simulink model "StateObserver_4"  (Simulink 8.3)
settings: configuration reference "mpc555rt_ref_debug_config" (kept outside this file)
values from neighbouring files (symbols this model uses):
  dt = 0.0192307692308    [newvars_4_25.mat]
  g = 32.174    [newvars_4_25.mat]
  HD0noaa = 48.3774    [newvars_4_25.mat]
  HE0noaa = 0.8962    [newvars_4_25.mat]
  HN0noaa = 20.6483    [newvars_4_25.mat]
  P0_est_sta = [100 0 0 0 0 0 0 0 0 0 0 0 ... (225 elements, 15x15)]    [newvars_4_25.mat]
  Q_obs_sta = [0.001 0 0 0 0 0 0 0 0 0 0 0 ... (225 elements, 15x15)]    [newvars_4_25.mat]
  R_obs_sta = [1 0 0 0 0 0 0 0 0 0 0.01 0 ... (81 elements, 9x9)]    [newvars_4_25.mat]
  saturation_max_sta = [1 0.261799387799 0.349065850399 0.174532925199 200 1.57079632679 1.57079632679 3.14159265359 3.14159265359 inf 15.7079632679 15.7079632679 ... (15 elements, 1x15)]    [newvars_4_25.mat]
  saturation_min_sta = [0.15 -0.261799387799 -0.349065850399 -0.174532925199 2.22044604925e-15 -1.57079632679 -1.57079632679 -3.14159265359 -3.14159265359 -inf -15.7079632679 -15.7079632679 ... (15 elements, 1x15)]    [newvars_4_25.mat]
  x0_est_sta = [0.55 0.0200712863979 0 0 45.808269954 -0.00604049793249 0 0 -0.00232644648767 0 0 -6.36434657562e-08 ... (15 elements, 15x1)]    [newvars_4_25.mat]
settings Model: Creator=Rick Riley  LastModifiedBy=gonzalo
settings ConfigSet: SourceName=mpc555rt_ref_debug_config  SourceLocation=Base Workspace

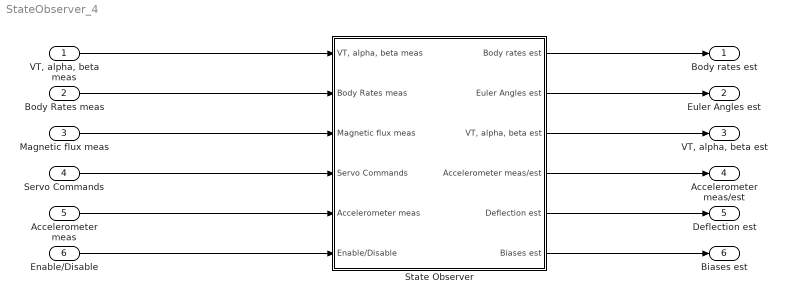
== system StateObserver_4 ==
  "VT, alpha, beta meas" : Inport  OutDataTypeStr=Bus: VT_A_B_bus  SampleTime=dt  BusOutputAsStruct=on
  Body Rates meas : Inport  Port=2  OutDataTypeStr=Bus: INS_rates_bus  SampleTime=dt
  Magnetic flux meas : Inport  Port=3  OutDataTypeStr=Bus: MagnetometerFlux
  Servo Commands : Inport  Port=4  OutDataTypeStr=Bus: Control_cmd_bus
  Accelerometer meas : Inport  Port=5  OutDataTypeStr=Bus: Accelerometer
  Enable/Disable : Inport  Port=6  OutDataTypeStr=boolean  SampleTime=dt
  State Observer : Subsystem
  Body rates est : Outport  OutDataTypeStr=Bus: INS_rates_bus  BusOutputAsStruct=on
  Euler Angles est : Outport  Port=2  OutDataTypeStr=Bus: INS_angles_bus  BusOutputAsStruct=on
  "VT, alpha, beta est" : Outport  Port=3  OutDataTypeStr=Bus: VT_A_B_bus  BusOutputAsStruct=on
  Accelerometer meas/est : Outport  Port=4  OutDataTypeStr=Bus: Accelerometer  BusOutputAsStruct=on
  Deflection est : Outport  Port=5  OutDataTypeStr=Bus: ControlSurfaceDeflections  BusOutputAsStruct=on
  Biases est : Outport  Port=6  BusOutputAsStruct=on
  wires:
  "VT, alpha, beta meas"/1 -> State Observer/1("VT, alpha, beta meas")
  Body Rates meas/1 -> State Observer/2(Body Rates meas)
  State Observer/3("VT, alpha, beta est") -> "VT, alpha, beta est"/1
  State Observer/1(Body rates est) -> Body rates est/1
  State Observer/2(Euler Angles est) -> Euler Angles est/1
  State Observer/4(Accelerometer meas/est) -> Accelerometer meas/est/1
  Enable/Disable/1 -> State Observer/6(Enable/Disable)
  State Observer/5(Deflection est) -> Deflection est/1
  State Observer/6(Biases est) -> Biases est/1
  Magnetic flux meas/1 -> State Observer/3(Magnetic flux meas)
  Servo Commands/1 -> State Observer/4(Servo Commands)
  Accelerometer meas/1 -> State Observer/5(Accelerometer meas)

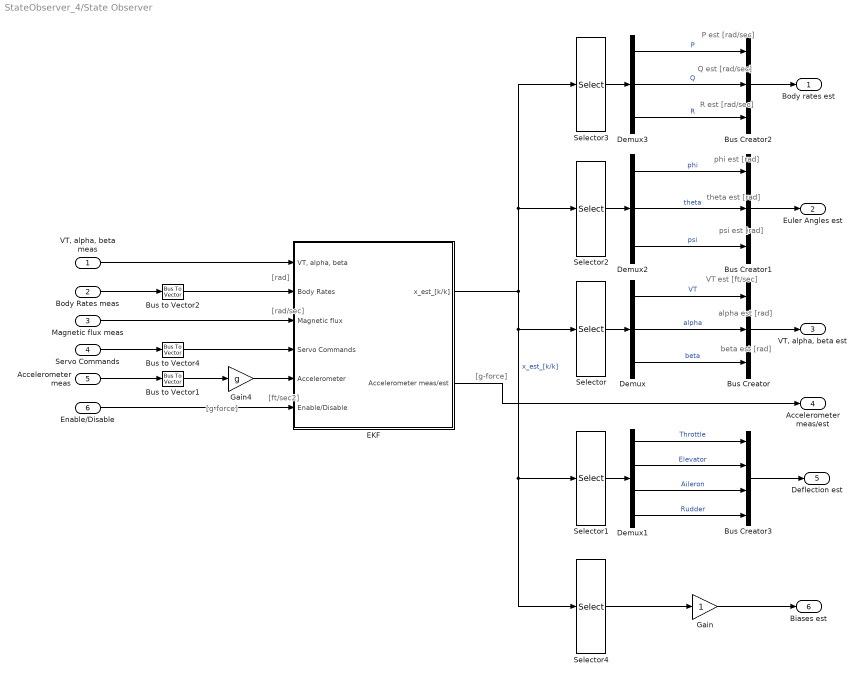
== system StateObserver_4/State Observer ==
  note: alpha est [rad]
  note: beta est [rad]
  note: VT est [ft/sec]
  note: Q est [rad/sec]
  note: R est [rad/sec]
  note: P est [rad/sec]
  note: phi est [rad]
  note: theta est [rad]
  note: [ft/sec2]
  note: [g-force]
  note: [rad/sec]
  note: [rad]
  note: psi est [rad]
  note: [g-force]
  "VT, alpha, beta meas" : Inport
  Body Rates meas : Inport  Port=2  OutDataTypeStr=Bus: INS_rates_bus  SampleTime=dt
  Magnetic flux meas : Inport  Port=3  OutDataTypeStr=Bus: MagnetometerFlux
  Servo Commands : Inport  Port=4  OutDataTypeStr=Bus: Control_cmd_bus  BusOutputAsStruct=on
  Accelerometer meas : Inport  Port=5  OutDataTypeStr=Bus: Accelerometer
  Enable/Disable : Inport  Port=6  OutDataTypeStr=boolean  SampleTime=dt
  Bus Creator : BusCreator  Inputs=3  OutDataTypeStr=Bus: VT_A_B_bus  NonVirtualBus=on
  Bus Creator1 : BusCreator  Inputs=3  OutDataTypeStr=Bus: INS_angles_bus  NonVirtualBus=on
  Bus Creator2 : BusCreator  Inputs=3  OutDataTypeStr=Bus: INS_rates_bus  NonVirtualBus=on
  Bus Creator3 : BusCreator  OutDataTypeStr=Bus: ControlSurfaceDeflections  NonVirtualBus=on
  Bus to Vector1 : BusToVector
  Bus to Vector2 : BusToVector
  Bus to Vector4 : BusToVector
  Demux : Demux  Outputs=3
  Demux1 : Demux
  Demux2 : Demux  Outputs=3
  Demux3 : Demux  Outputs=3
  EKF : Subsystem
  Gain : Gain
  Gain4 : Gain  Gain=g
  Selector : Selector  InputPortWidth=15  Indices=[5 6 7]
  Selector1 : Selector  InputPortWidth=15  Indices=[1 2 3 4]
  Selector2 : Selector  InputPortWidth=15  Indices=[8 9 10]
  Selector3 : Selector  InputPortWidth=15  Indices=[11 12 13]
  Selector4 : Selector  InputPortWidth=15  Indices=[14 15]
  Body rates est : Outport  OutDataTypeStr=Bus: INS_rates_bus
  Euler Angles est : Outport  Port=2  OutDataTypeStr=Bus: INS_angles_bus  BusOutputAsStruct=on
  "VT, alpha, beta est" : Outport  Port=3  OutDataTypeStr=Bus: VT_A_B_bus
  Accelerometer meas/est : Outport  Port=4  OutDataTypeStr=Bus: Accelerometer  BusOutputAsStruct=on
  Deflection est : Outport  Port=5  OutDataTypeStr=Bus: ControlSurfaceDeflections  BusOutputAsStruct=on
  Biases est : Outport  Port=6  BusOutputAsStruct=on
  wires:
  Bus Creator/1 -> "VT, alpha, beta est"/1
  Demux/1 -> Bus Creator/1  "VT"
  Demux/2 -> Bus Creator/2  "alpha"
  Demux/3 -> Bus Creator/3  "beta"
  Selector/1 -> Demux/1
  Selector2/1 -> Demux2/1
  Demux2/1 -> Bus Creator1/1  "phi"
  Demux2/2 -> Bus Creator1/2  "theta"
  Bus Creator1/1 -> Euler Angles est/1
  Bus Creator2/1 -> Body rates est/1
  Demux3/1 -> Bus Creator2/1  "P"
  Demux3/2 -> Bus Creator2/2  "Q"
  Demux3/3 -> Bus Creator2/3  "R"
  Selector3/1 -> Demux3/1
  Bus to Vector1/1 -> Gain4/1
  Accelerometer meas/1 -> Bus to Vector1/1
  Body Rates meas/1 -> Bus to Vector2/1
  Bus to Vector2/1 -> EKF/2(Body Rates)
  Gain4/1 -> EKF/5(Accelerometer)
  "VT, alpha, beta meas"/1 -> EKF/1("VT, alpha, beta")
  Servo Commands/1 -> Bus to Vector4/1
  Demux2/3 -> Bus Creator1/3  "psi"
  EKF/2(Accelerometer meas/est) -> Accelerometer meas/est/1
  Enable/Disable/1 -> EKF/6(Enable/Disable)
  Selector1/1 -> Demux1/1
  Demux1/4 -> Bus Creator3/4  "Rudder"
  Demux1/2 -> Bus Creator3/2  "Elevator"
  Demux1/3 -> Bus Creator3/3  "Aileron"
  Demux1/1 -> Bus Creator3/1  "Throttle"
  Bus Creator3/1 -> Deflection est/1
  EKF/1(x_est_[k/k]) -> Selector3/1, Selector2/1, Selector/1, Selector1/1, Selector4/1  "x_est_[k/k]"
  Selector4/1 -> Gain/1
  Gain/1 -> Biases est/1
  Magnetic flux meas/1 -> EKF/3(Magnetic flux)
  Bus to Vector4/1 -> EKF/4(Servo Commands)

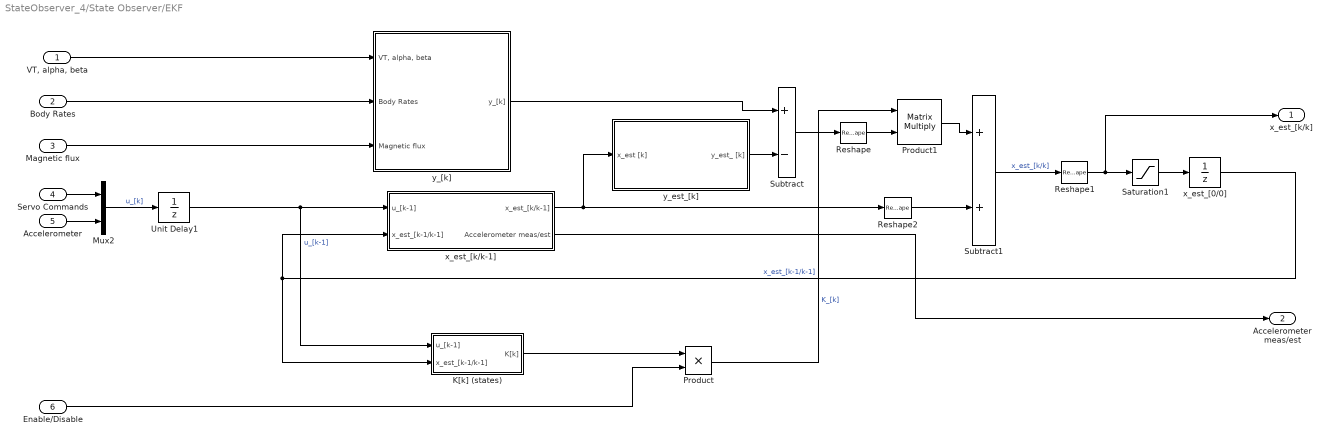
== system StateObserver_4/State Observer/EKF ==
  "VT, alpha, beta" : Inport  OutDataTypeStr=Bus: VT_A_B_bus
  Body Rates : Inport  Port=2  SampleTime=dt
  Magnetic flux : Inport  Port=3  OutDataTypeStr=Bus: MagnetometerFlux
  Servo Commands : Inport  Port=4
  Accelerometer : Inport  Port=5
  Enable/Disable : Inport  Port=6  OutDataTypeStr=boolean  SampleTime=dt
  K[k] (states) : Subsystem
  Mux2 : Mux  Inputs=2
  Product : Product  RndMeth=Zero
  Product1 : Product  Multiplication=Matrix(*)  RndMeth=Zero
  Reshape : Reshape  OutputDimensionality=Column vector (2-D)
  Reshape1 : Reshape
  Reshape2 : Reshape  OutputDimensionality=Column vector (2-D)
  Saturation1 : Saturate  UpperLimit=saturation_max_sta  LowerLimit=saturation_min_sta
  Subtract : Sum  Inputs=+-
  Subtract1 : Sum
  Unit Delay1 : UnitDelay  SampleTime=dt
  x_est_[0/0] : UnitDelay  InitialCondition=x0_est_sta  SampleTime=dt
  x_est_[k/k-1] : Subsystem
  y_[k] : Subsystem
  y_est_[k] : Subsystem
  x_est_[k/k] : Outport
  Accelerometer meas/est : Outport  Port=2  OutDataTypeStr=Bus: Accelerometer  BusOutputAsStruct=on
  wires:
  y_[k]/1(y_[k]) -> Subtract/1
  "VT, alpha, beta"/1 -> y_[k]/1("VT, alpha, beta")
  Subtract1/1 -> Reshape1/1  "x_est_[k/k]"
  x_est_[0/0]/1 -> K[k] (states)/2(x_est_[k-1/k-1]), x_est_[k/k-1]/2(x_est_[k-1/k-1])  "x_est_[k-1/k-1]"
  Unit Delay1/1 -> K[k] (states)/1(u_[k-1]), x_est_[k/k-1]/1(u_[k-1])  "u_[k-1]"
  Saturation1/1 -> x_est_[0/0]/1
  y_est_[k]/1(y_est_ [k]) -> Subtract/2
  Product/1 -> Product1/1  "K_[k]"
  Product1/1 -> Subtract1/1
  Mux2/1 -> Unit Delay1/1  "u_[k]"
  Accelerometer/1 -> Mux2/2
  Servo Commands/1 -> Mux2/1
  Body Rates/1 -> y_[k]/2(Body Rates)
  Subtract/1 -> Reshape/1
  x_est_[k/k-1]/1(x_est_[k/k-1]) -> Reshape2/1, y_est_[k]/1(x_est [k])
  x_est_[k/k-1]/2(Accelerometer meas/est) -> Accelerometer meas/est/1
  K[k] (states)/1(K[k]) -> Product/1
  Enable/Disable/1 -> Product/2
  Reshape/1 -> Product1/2
  Reshape1/1 -> Saturation1/1, x_est_[k/k]/1
  Reshape2/1 -> Subtract1/2
  Magnetic flux/1 -> y_[k]/3(Magnetic flux)

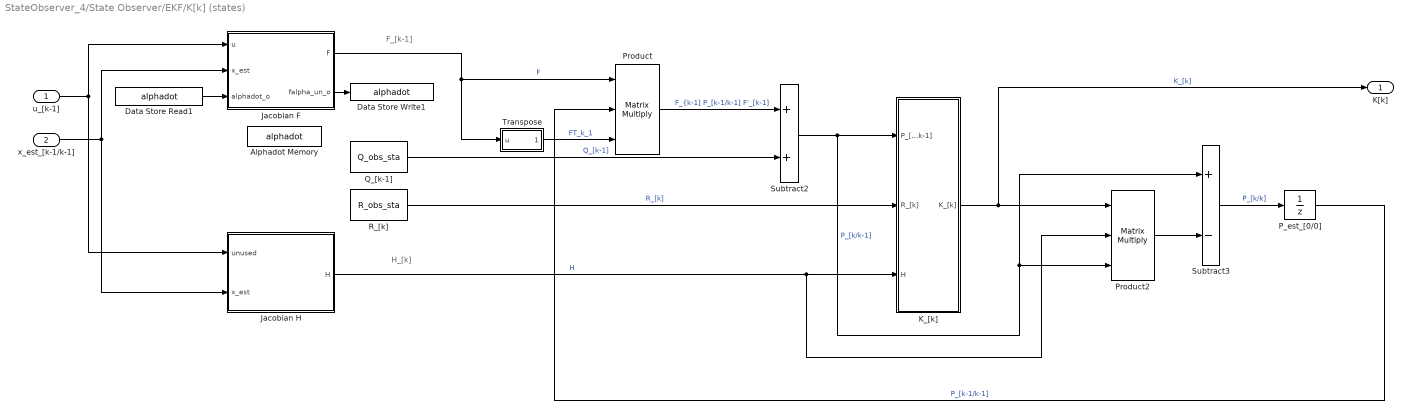
== system StateObserver_4/State Observer/EKF/K[k] (states) ==
  note: H_[k]
  note: F_[k-1]
  u_[k-1] : Inport
  x_est_[k-1/k-1] : Inport  Port=2
  Alphadot Memory : DataStoreMemory  DataStoreName=alphadot  ReadBeforeWriteMsg=warning  WriteAfterWriteMsg=warning  WriteAfterReadMsg=warning  OutDataTypeStr=double
  Data Store Read1 : DataStoreRead  DataStoreName=alphadot  SampleTime=dt
  Data Store Write1 : DataStoreWrite  DataStoreName=alphadot
  Jacobian F : MATLAB Function  TreatAsAtomicUnit=on
  Jacobian H : MATLAB Function  TreatAsAtomicUnit=on
  K_[k] : Subsystem
  P_est_[0/0] : UnitDelay  InitialCondition=P0_est_sta  SampleTime=dt
  Product : Product  Inputs=3  Multiplication=Matrix(*)  RndMeth=Zero
  Product2 : Product  Inputs=3  Multiplication=Matrix(*)  RndMeth=Zero
  Q_[k-1] : Constant  Value=Q_obs_sta
  R_[k] : Constant  Value=R_obs_sta
  Subtract2 : Sum
  Subtract3 : Sum  Inputs=+-
  Transpose : MATLAB Function  TreatAsAtomicUnit=on
  K[k] : Outport
  wires:
  K_[k]/1(K_[k]) -> K[k]/1, Product2/1  "K_[k]"
  x_est_[k-1/k-1]/1 -> Jacobian F/2(x_est), Jacobian H/2(x_est)
  u_[k-1]/1 -> Jacobian F/1(u), Jacobian H/1(unused)
  Jacobian F/1(F) -> Transpose/1(u), Product/1  "F"
  P_est_[0/0]/1 -> Product/2  "P_[k-1/k-1]"
  Subtract3/1 -> P_est_[0/0]/1  "P_[k/k]"
  Product2/1 -> Subtract3/2
  R_[k]/1 -> K_[k]/2(R_[k])  "R_[k]"
  Jacobian H/1(H) -> Product2/2, K_[k]/3(H)  "H"
  Subtract2/1 -> Product2/3, Subtract3/1, K_[k]/1(P_[k/k-1])  "P_[k/k-1]"
  Q_[k-1]/1 -> Subtract2/2  "Q_[k-1]"
  Product/1 -> Subtract2/1  "F_{k-1] P_[k-1/k-1] F'_[k-1]"
  Transpose/1(FT_k_1) -> Product/3  "FT_k_1"
  Data Store Read1/1 -> Jacobian F/3(alphadot_o)
  Jacobian F/2(falpha_un_o) -> Data Store Write1/1

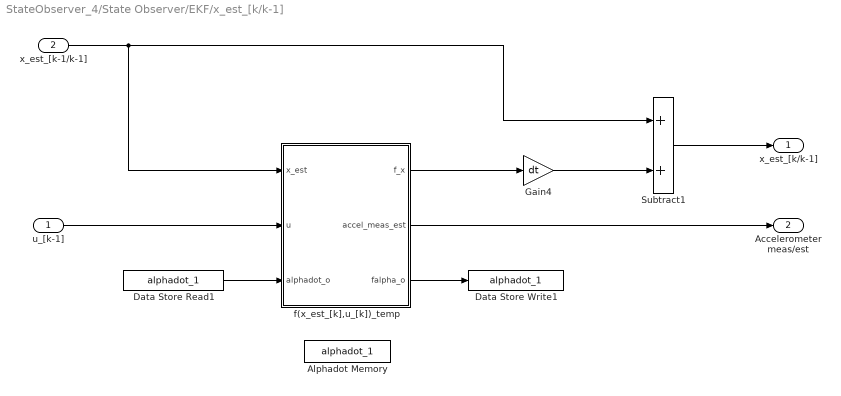
== system StateObserver_4/State Observer/EKF/x_est_[k/k-1] ==
  u_[k-1] : Inport
  x_est_[k-1/k-1] : Inport  Port=2
  Alphadot Memory : DataStoreMemory  DataStoreName=alphadot_1  ReadBeforeWriteMsg=warning  WriteAfterWriteMsg=warning  WriteAfterReadMsg=warning  OutDataTypeStr=double
  Data Store Read1 : DataStoreRead  DataStoreName=alphadot_1  SampleTime=dt
  Data Store Write1 : DataStoreWrite  DataStoreName=alphadot_1
  Gain4 : Gain  Gain=dt
  Subtract1 : Sum
  f(x_est_[k],u_[k])_temp : MATLAB Function  TreatAsAtomicUnit=on
  x_est_[k/k-1] : Outport
  Accelerometer meas/est : Outport  Port=2  OutDataTypeStr=Bus: Accelerometer  BusOutputAsStruct=on
  wires:
  Gain4/1 -> Subtract1/2
  x_est_[k-1/k-1]/1 -> Subtract1/1, f(x_est_[k],u_[k])_temp/1(x_est)
  u_[k-1]/1 -> f(x_est_[k],u_[k])_temp/2(u)
  Subtract1/1 -> x_est_[k/k-1]/1
  f(x_est_[k],u_[k])_temp/1(f_x) -> Gain4/1
  f(x_est_[k],u_[k])_temp/2(accel_meas_est) -> Accelerometer meas/est/1
  f(x_est_[k],u_[k])_temp/3(falpha_o) -> Data Store Write1/1
  Data Store Read1/1 -> f(x_est_[k],u_[k])_temp/3(alphadot_o)

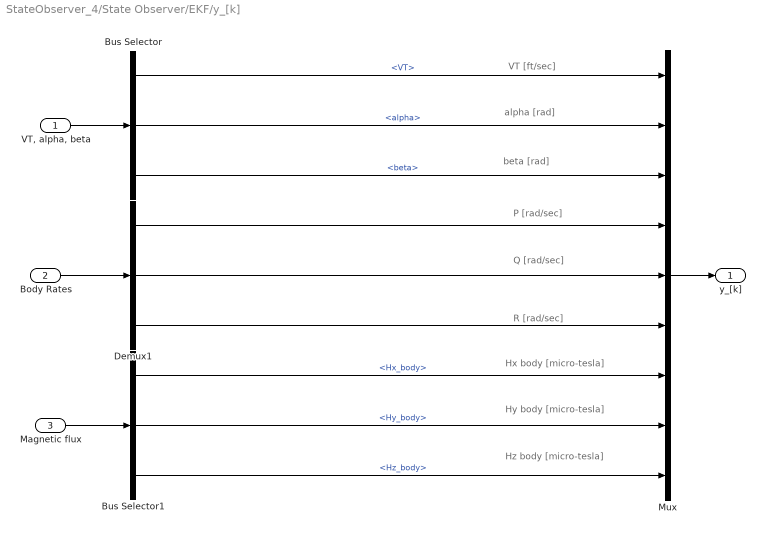
== system StateObserver_4/State Observer/EKF/y_[k] ==
  note: Hz body [micro-tesla]
  note: Hy body [micro-tesla]
  note: Hx body [micro-tesla]
  note: beta [rad]
  note: alpha [rad]
  note: VT [ft/sec]
  note: R [rad/sec]
  note: Q [rad/sec]
  note: P [rad/sec]
  "VT, alpha, beta" : Inport
  Body Rates : Inport  Port=2  SampleTime=dt
  Magnetic flux : Inport  Port=3  OutDataTypeStr=Bus: MagnetometerFlux
  Bus Selector : BusSelector  OutputSignals=VT,alpha,beta
  Bus Selector1 : BusSelector  OutputSignals=Hx_body,Hy_body,Hz_body
  Demux1 : Demux  Outputs=3
  Mux : Mux  Inputs=9
  y_[k] : Outport
  wires:
  "VT, alpha, beta"/1 -> Bus Selector/1
  Demux1/2 -> Mux/5
  Demux1/3 -> Mux/6
  Demux1/1 -> Mux/4
  Mux/1 -> y_[k]/1
  Bus Selector/3 -> Mux/3  "<beta>"
  Bus Selector/2 -> Mux/2  "<alpha>"
  Bus Selector/1 -> Mux/1  "<VT>"
  Body Rates/1 -> Demux1/1
  Magnetic flux/1 -> Bus Selector1/1
  Bus Selector1/3 -> Mux/9  "<Hz_body>"
  Bus Selector1/1 -> Mux/7  "<Hx_body>"
  Bus Selector1/2 -> Mux/8  "<Hy_body>"

== system StateObserver_4/State Observer/EKF/y_est_[k] ==
  x_est [k] : Inport
  h(x_est_[k],u_[k]) : Subsystem
  y_est_ [k] : Outport
  wires:
  x_est [k]/1 -> h(x_est_[k],u_[k])/1(x_est [k])
  h(x_est_[k],u_[k])/1(y_est_ [k]) -> y_est_ [k]/1

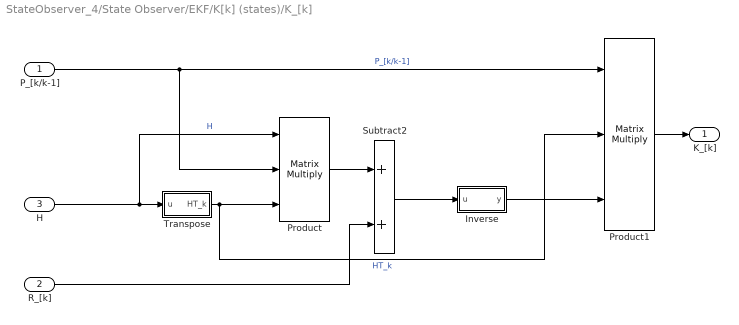
== system StateObserver_4/State Observer/EKF/K[k] (states)/K_[k] ==
  P_[k/k-1] : Inport
  R_[k] : Inport  Port=2
  H : Inport  Port=3
  Inverse : MATLAB Function  TreatAsAtomicUnit=on
  Product : Product  Inputs=3  Multiplication=Matrix(*)  RndMeth=Zero
  Product1 : Product  Inputs=3  Multiplication=Matrix(*)  RndMeth=Zero
  Subtract2 : Sum
  Transpose : MATLAB Function  TreatAsAtomicUnit=on
  K_[k] : Outport
  wires:
  Inverse/1(y) -> Product1/3
  Product1/1 -> K_[k]/1
  Subtract2/1 -> Inverse/1(u)
  R_[k]/1 -> Subtract2/2
  Product/1 -> Subtract2/1
  Transpose/1(HT_k) -> Product1/2, Product/3  "HT_k"
  P_[k/k-1]/1 -> Product1/1, Product/2  "P_[k/k-1]"
  H/1 -> Transpose/1(u), Product/1  "H"

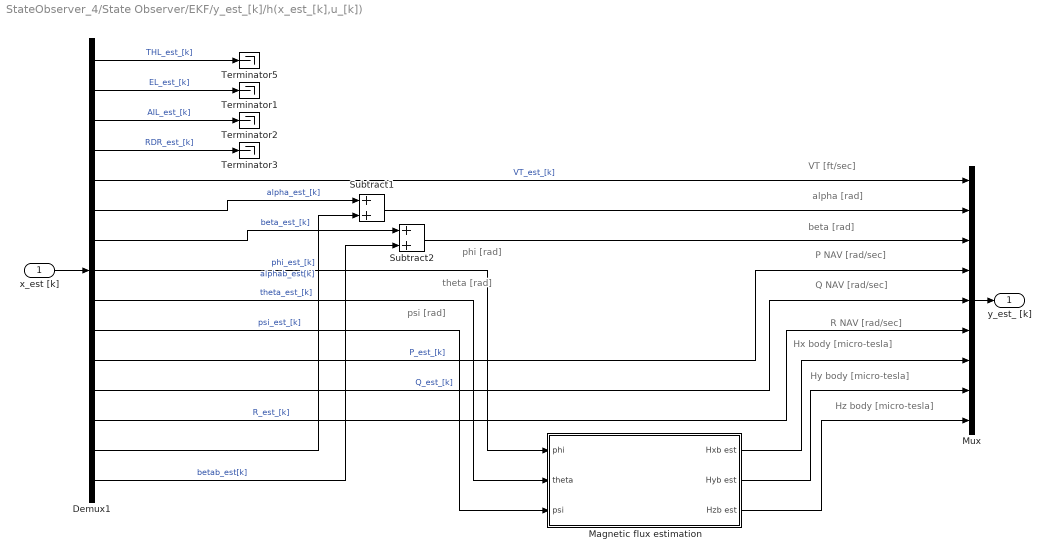
== system StateObserver_4/State Observer/EKF/y_est_[k]/h(x_est_[k],u_[k]) ==
  note: psi [rad]
  note: Hz body [micro-tesla]
  note: Hy body [micro-tesla]
  note: Hx body [micro-tesla]
  note: phi [rad]
  note: theta [rad]
  note: beta [rad]
  note: alpha [rad]
  note: VT [ft/sec]
  note: P NAV [rad/sec]
  note: Q NAV [rad/sec]
  note: R NAV [rad/sec]
  x_est [k] : Inport
  Demux1 : Demux  Outputs=15
  Magnetic flux estimation : Subsystem
  Mux : Mux  Inputs=9
  Subtract1 : Sum
  Subtract2 : Sum
  Terminator{1..3,5} (4 alike) : Terminator
  y_est_ [k] : Outport
  wires:
  Demux1/4 -> Terminator3/1  "RDR_est_[k]"
  Demux1/3 -> Terminator2/1  "AIL_est_[k]"
  Demux1/2 -> Terminator1/1  "EL_est_[k]"
  Demux1/1 -> Terminator5/1  "THL_est_[k]"
  x_est [k]/1 -> Demux1/1
  Demux1/14 -> Subtract1/2  "alphab_est[k]"
  Demux1/15 -> Subtract2/2  "betab_est[k]"
  Demux1/5 -> Mux/1  "VT_est_[k]"
  Demux1/6 -> Subtract1/1  "alpha_est_[k]"
  Demux1/7 -> Subtract2/1  "beta_est_[k]"
  Demux1/8 -> Magnetic flux estimation/1(phi)  "phi_est_[k]"
  Demux1/9 -> Magnetic flux estimation/2(theta)  "theta_est_[k]"
  Demux1/11 -> Mux/4  "P_est_[k]"
  Demux1/12 -> Mux/5  "Q_est_[k]"
  Demux1/13 -> Mux/6  "R_est_[k]"
  Subtract1/1 -> Mux/2
  Subtract2/1 -> Mux/3
  Mux/1 -> y_est_ [k]/1
  Magnetic flux estimation/2(Hyb est) -> Mux/8
  Magnetic flux estimation/3(Hzb est) -> Mux/9
  Magnetic flux estimation/1(Hxb est) -> Mux/7
  Demux1/10 -> Magnetic flux estimation/3(psi)  "psi_est_[k]"

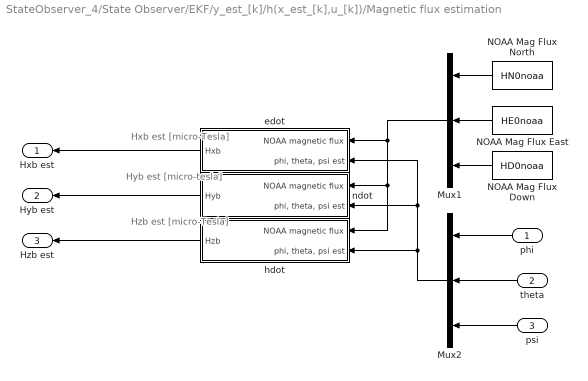
== system StateObserver_4/State Observer/EKF/y_est_[k]/h(x_est_[k],u_[k])/Magnetic flux estimation ==
  note: Hxb est [micro-Tesla]
  note: Hzb est [micro-Tesla]
  note: Hyb est [micro-tesla]
  phi : Inport
  theta : Inport  Port=2
  psi : Inport  Port=3
  Mux1 : Mux  Inputs=3
  Mux2 : Mux  Inputs=3
  NOAA Mag Flux Down : Constant  Value=HD0noaa
  NOAA Mag Flux East : Constant  Value=HE0noaa
  NOAA Mag Flux North : Constant  Value=HN0noaa
  edot : Subsystem
  hdot : Subsystem
  ndot : Subsystem
  Hxb est : Outport
  Hyb est : Outport  Port=2
  Hzb est : Outport  Port=3
  wires:
  hdot/1(Hzb) -> Hzb est/1
  edot/1(Hxb) -> Hxb est/1
  ndot/1(Hyb) -> Hyb est/1
  Mux1/1 -> edot/1(NOAA magnetic flux), ndot/1(NOAA magnetic flux), hdot/1(NOAA magnetic flux)
  NOAA Mag Flux North/1 -> Mux1/1
  NOAA Mag Flux East/1 -> Mux1/2
  NOAA Mag Flux Down/1 -> Mux1/3
  Mux2/1 -> hdot/2("phi, theta, psi est"), ndot/2("phi, theta, psi est"), edot/2("phi, theta, psi est")
  phi/1 -> Mux2/1
  theta/1 -> Mux2/2
  psi/1 -> Mux2/3

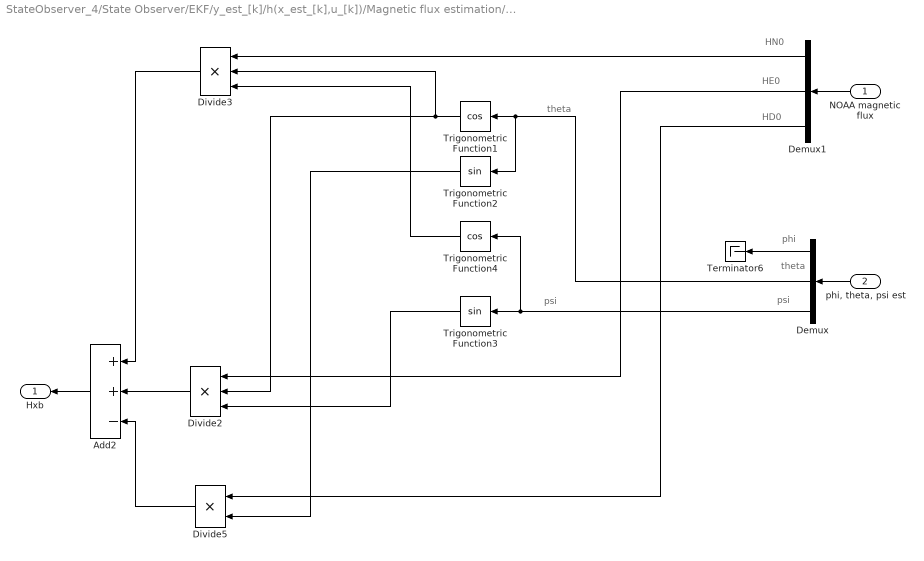
== system StateObserver_4/State Observer/EKF/y_est_[k]/h(x_est_[k],u_[k])/Magnetic flux estimation/edot ==
  note: phi
  note: theta
  note: psi
  note: theta
  note: psi
  note: HN0
  note: HE0
  note: HD0
  NOAA magnetic flux : Inport
  "phi, theta, psi est" : Inport  Port=2
  Add2 : Sum  Inputs=++-
  Demux : Demux  Outputs=3
  Demux1 : Demux  Outputs=3
  Divide2 : Product  Inputs=***
  Divide3 : Product  Inputs=***
  Divide5 : Product  Inputs=**
  Terminator6 : Terminator
  Trigonometric Function1 : Trigonometry  Operator=cos
  Trigonometric Function2 : Trigonometry
  Trigonometric Function3 : Trigonometry
  Trigonometric Function4 : Trigonometry  Operator=cos
  Hxb : Outport
  wires:
  Divide5/1 -> Add2/3
  Divide2/1 -> Add2/2
  Divide3/1 -> Add2/1
  Add2/1 -> Hxb/1
  Trigonometric Function3/1 -> Divide2/3
  Trigonometric Function4/1 -> Divide3/3
  Trigonometric Function1/1 -> Divide3/2, Divide2/2
  "phi, theta, psi est"/1 -> Demux/1
  Demux/2 -> Trigonometric Function2/1, Trigonometric Function1/1
  Demux/3 -> Trigonometric Function3/1, Trigonometric Function4/1
  NOAA magnetic flux/1 -> Demux1/1
  Demux1/1 -> Divide3/1
  Demux1/2 -> Divide2/1
  Demux1/3 -> Divide5/1
  Trigonometric Function2/1 -> Divide5/2
  Demux/1 -> Terminator6/1

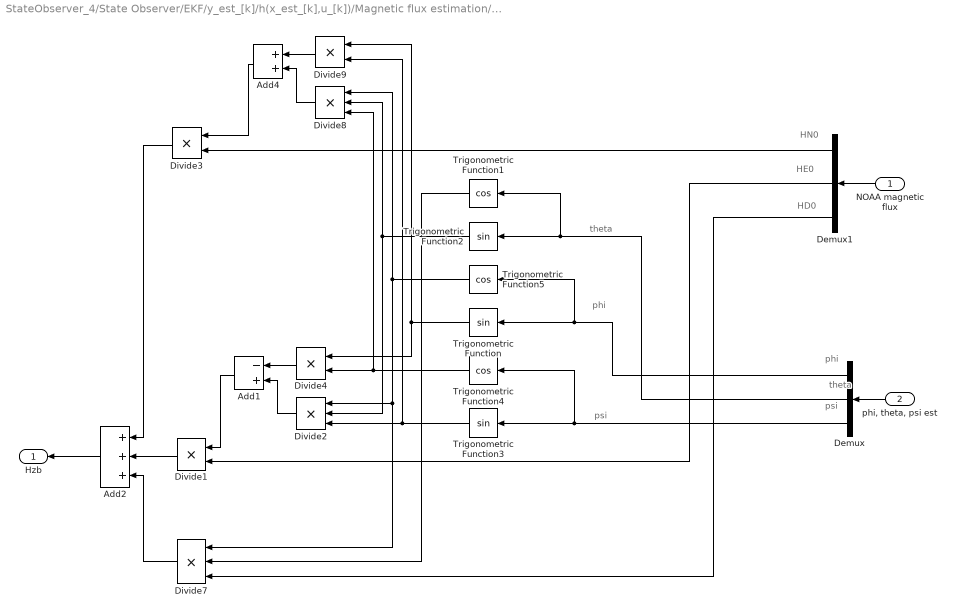
== system StateObserver_4/State Observer/EKF/y_est_[k]/h(x_est_[k],u_[k])/Magnetic flux estimation/hdot ==
  note: phi
  note: theta
  note: psi
  note: HN0
  note: HE0
  note: HD0
  note: theta
  note: phi
  note: psi
  NOAA magnetic flux : Inport
  "phi, theta, psi est" : Inport  Port=2
  Add1 : Sum  Inputs=-+
  Add2 : Sum  Inputs=+++
  Add4 : Sum
  Demux : Demux  Outputs=3
  Demux1 : Demux  Outputs=3
  Divide{1,3..4,9} (4 alike) : Product  Inputs=**
  Divide2 : Product  Inputs=***
  Divide7 : Product  Inputs=***
  Divide8 : Product  Inputs=***
  Trigonometric Function : Trigonometry
  Trigonometric Function1 : Trigonometry  Operator=cos
  Trigonometric Function2 : Trigonometry
  Trigonometric Function3 : Trigonometry
  Trigonometric Function4 : Trigonometry  Operator=cos
  Trigonometric Function5 : Trigonometry  Operator=cos
  Hzb : Outport
  wires:
  "phi, theta, psi est"/1 -> Demux/1
  NOAA magnetic flux/1 -> Demux1/1
  Demux1/1 -> Divide3/2
  Divide7/1 -> Add2/3
  Divide1/1 -> Add2/2
  Divide3/1 -> Add2/1
  Add2/1 -> Hzb/1
  Divide2/1 -> Add1/2
  Divide4/1 -> Add1/1
  Add1/1 -> Divide1/1
  Demux/1 -> Trigonometric Function/1, Trigonometric Function5/1
  Demux/2 -> Trigonometric Function2/1, Trigonometric Function1/1
  Demux/3 -> Trigonometric Function3/1, Trigonometric Function4/1
  Divide8/1 -> Add4/2
  Divide9/1 -> Add4/1
  Add4/1 -> Divide3/1
  Trigonometric Function/1 -> Divide9/1, Divide4/1
  Trigonometric Function3/1 -> Divide9/2, Divide2/3
  Trigonometric Function5/1 -> Divide8/1, Divide2/1, Divide7/1
  Trigonometric Function2/1 -> Divide8/2, Divide2/2
  Trigonometric Function4/1 -> Divide8/3, Divide4/2
  Demux1/2 -> Divide1/2
  Demux1/3 -> Divide7/3
  Trigonometric Function1/1 -> Divide7/2

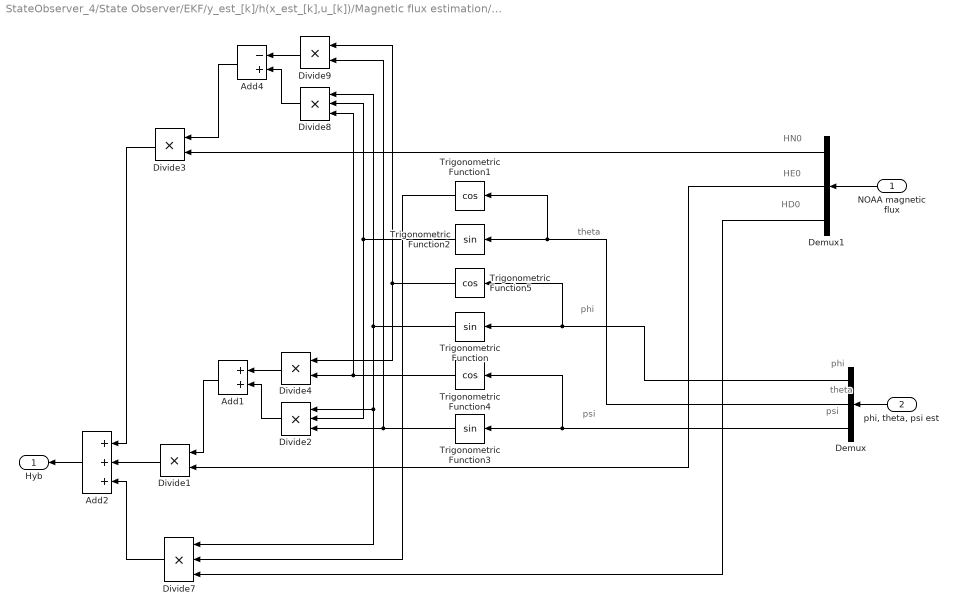
== system StateObserver_4/State Observer/EKF/y_est_[k]/h(x_est_[k],u_[k])/Magnetic flux estimation/ndot ==
  note: phi
  note: theta
  note: psi
  note: theta
  note: phi
  note: psi
  note: HN0
  note: HE0
  note: HD0
  NOAA magnetic flux : Inport
  "phi, theta, psi est" : Inport  Port=2
  Add1 : Sum
  Add2 : Sum  Inputs=+++
  Add4 : Sum  Inputs=-+
  Demux : Demux  Outputs=3
  Demux1 : Demux  Outputs=3
  Divide{1,3..4,9} (4 alike) : Product  Inputs=**
  Divide2 : Product  Inputs=***
  Divide7 : Product  Inputs=***
  Divide8 : Product  Inputs=***
  Trigonometric Function : Trigonometry
  Trigonometric Function1 : Trigonometry  Operator=cos
  Trigonometric Function2 : Trigonometry
  Trigonometric Function3 : Trigonometry
  Trigonometric Function4 : Trigonometry  Operator=cos
  Trigonometric Function5 : Trigonometry  Operator=cos
  Hyb : Outport
  wires:
  Divide7/1 -> Add2/3
  Divide1/1 -> Add2/2
  Divide3/1 -> Add2/1
  Add2/1 -> Hyb/1
  Divide2/1 -> Add1/2
  Divide4/1 -> Add1/1
  Add1/1 -> Divide1/1
  "phi, theta, psi est"/1 -> Demux/1
  Demux/1 -> Trigonometric Function/1, Trigonometric Function5/1
  Demux/2 -> Trigonometric Function2/1, Trigonometric Function1/1
  Demux/3 -> Trigonometric Function3/1, Trigonometric Function4/1
  NOAA magnetic flux/1 -> Demux1/1
  Demux1/1 -> Divide3/2
  Demux1/2 -> Divide1/2
  Demux1/3 -> Divide7/3
  Divide8/1 -> Add4/2
  Divide9/1 -> Add4/1
  Add4/1 -> Divide3/1
  Trigonometric Function5/1 -> Divide9/1, Divide4/1
  Trigonometric Function3/1 -> Divide9/2, Divide2/3
  Trigonometric Function/1 -> Divide8/1, Divide7/1, Divide2/1
  Trigonometric Function2/1 -> Divide8/2, Divide2/2
  Trigonometric Function4/1 -> Divide8/3, Divide4/2
  Trigonometric Function1/1 -> Divide7/2

== matlab function State Observer/EKF/K[k] (states)/K_[k]/Inverse ==
  data: u input double; y output double
function y = fcn(u)
%#codegen

y = u^-1;

== matlab function State Observer/EKF/x_est_[k//k-1]/f(x_est_[k],u_[k])_temp ==
  data: x_est input double; u input double; alphadot_o input double; f_x output double; accel_meas_est output Bus: Accelerometer size=1; rho parameter double; S parameter double; Cbar parameter double; b parameter double; weight parameter double; g parameter double; IxxB parameter double; IyyB parameter double; IzzB parameter double; IxzB parameter double; CD0 parameter double; CDu parameter double; CDa parameter double; CDq parameter double; CDadot parameter double; CDde parameter double; CD0_bar parameter double; Cyb parameter double; Cyp parameter double; Cyr parameter double; Cyda parameter double; Cydr parameter double; CL0 parameter double; CLa parameter double; CLq parameter double; CLadot parameter double; CLu parameter double; CLde parameter double; Clb parameter double; Clp parameter double; Clr parameter double; Clda parameter double; Cldr parameter double; Cm0 parameter double; Cma parameter double; Cmq parameter double; Cmadot parameter double; Cmu parameter double; Cmde parameter double; Cnb parameter double; Cnp parameter double; Cnr parameter double; Cnda parameter double; Cndr parameter double; xT0 parameter double; xT1 parameter double; xT2 parameter double; Ptrim parameter double; Qtrim parameter double; Rtrim parameter double; Utrim parameter double; Athrottle parameter double; Bthrottle parameter double; Aelevator parameter double; Belevator parameter double; Aaileron parameter double; Baileron parameter double; Arudder parameter double; Brudder parameter double; ThrottleMax parameter double; ThrottleMin parameter double; ElevatorMax parameter double; ElevatorMin parameter double; AileronMax parameter double; AileronMin parameter double; RudderMax parameter double; RudderMin parameter double; falpha_o output double
function [f_x,...
          accel_meas_est,...
          falpha_o...
          ]=...
          f_x_u(x_est,...
                u,...
                alphadot_o,...
                rho,...
                S,Cbar,b,weight,g,IxxB,IyyB,IzzB,IxzB,...
                CD0,CDu,CDa,CDq,CDadot,CDde,...
                CD0_bar,...
                Cyb,Cyp,Cyr,Cyda,Cydr,...
                CL0,CLa,CLq,CLadot,CLu,CLde,...
                Clb,Clp,Clr,Clda,Cldr,...
                Cm0,Cma,Cmq,Cmadot,Cmu,Cmde,...
                Cnb,Cnp,Cnr,Cnda,Cndr,...
                xT0,xT1,xT2,...
                Ptrim,Qtrim,Rtrim,Utrim,...
                Athrottle,Bthrottle,...
                Aelevator,Belevator,...
                Aaileron,Baileron,...
                Arudder,Brudder,...
                ThrottleMax,ThrottleMin,...
                ElevatorMax,ElevatorMin,...
                AileronMax,AileronMin,...
                RudderMax,RudderMin)
          
%#codegen

THL_o=x_est(1);      %[-]
EL_o=x_est(2);       %[rad]
AIL_o=x_est(3);      %[rad]
RDR_o=x_est(4);      %[rad]
VT_o=x_est(5);       %[[ft/s]
alpha_o=x_est(6);    %[rad]
beta_o=x_est(7);     %[rad]
phi_o=x_est(8);      %[rad]
theta_o=x_est(9);    %[rad]
psi_o=x_est(10);     %[rad]
P_o=x_est(11);       %[rad/s]
Q_o=x_est(12);       %[rad/s]
R_o=x_est(13);       %[rad/s]
alphab_o=x_est(14);  %[rad]
betab_o=x_est(15);   %[rad]

THLcmd_o=u(1);       %[-]
ELcmd_o=u(2);        %[rad]
AILcmd_o=u(3);       %[rad]
RDRcmd_o=u(4);       %[rad]
accelX_meas_o=u(5);  %[ft/s2]
accelY_meas_o=u(6);  %[ft/s2]
accelZ_meas_o=u(7);  %[ft/s2]

[fTHL_o,fEL_o,fAIL_o,fRDR_o,...
 fVT_o,falpha_o,fbeta_o,fphi_o,ftheta_o,fpsi_o,fP_o,fQ_o,fR_o,...
 falphab_o,fbetab_o,...
 accelX_meas_est_o,accelY_meas_est_o,accelZ_meas_est_o...
 ]...
 =f_x_u_state_EKF_sailplane(...
                    alphadot_o,...
                    THL_o,EL_o,AIL_o,RDR_o,...
                    VT_o,alpha_o,beta_o,phi_o,theta_o,psi_o,P_o,Q_o,R_o,...
                    alphab_o,betab_o,...
                    THLcmd_o,ELcmd_o,AILcmd_o,RDRcmd_o,...
                    accelX_meas_o,accelY_meas_o,accelZ_meas_o,...
                    rho,...
                    S,Cbar,b,weight,g,IxxB,IyyB,IzzB,IxzB,...
                    CD0,CDu,CDa,CDq,CDadot,CDde,...
                    CD0_bar,...
                    Cyb,Cyp,Cyr,Cyda,Cydr,...
                    CL0,CLa,CLq,CLadot,CLu,CLde,...
                    Clb,Clp,Clr,Clda,Cldr,...
                    Cm0,Cma,Cmq,Cmadot,Cmu,Cmde,...
                    Cnb,Cnp,Cnr,Cnda,Cndr,...
                    xT0,xT1,xT2,...
                    Ptrim,Qtrim,Rtrim,Utrim,...
                    Athrottle,Bthrottle,...
                    Aelevator,Belevator,...
                    Aaileron,Baileron,...
                    Arudder,Brudder,...
                    ThrottleMax,ThrottleMin,...
                    ElevatorMax,ElevatorMin,...
                    AileronMax,AileronMin,...
                    RudderMax,RudderMin);

f_x=[fTHL_o;fEL_o;fAIL_o;fRDR_o;...
     fVT_o;falpha_o;fbeta_o;fphi_o;ftheta_o;fpsi_o;fP_o;fQ_o;fR_o;...
     falphab_o;fbetab_o];
 
accel_meas_est.Axb=accelX_meas_est_o/g; %[g-force]
accel_meas_est.Ayb=accelY_meas_est_o/g; %[g-force]
accel_meas_est.Azb=accelZ_meas_est_o/g; %[g-force]

== matlab function State Observer/EKF/K[k] (states)/Jacobian F ==
  data: u input double; F output double; x_est input double; alphadot_o input double; falpha_un_o output double; dt parameter double; rho parameter double; S parameter double; Cbar parameter double; b parameter double; weight parameter double; g parameter double; IxxB parameter double; IyyB parameter double; IzzB parameter double; IxzB parameter double; CD0 parameter double; CDu parameter double; CDa parameter double; CDq parameter double; CDadot parameter double; CDde parameter double; CD0_bar parameter double; Cyb parameter double; Cyp parameter double; Cyr parameter double; Cyda parameter double; Cydr parameter double; CL0 parameter double; CLa parameter double; CLq parameter double; CLadot parameter double; CLu parameter double; CLde parameter double; Clb parameter double; Clp parameter double; Clr parameter double; Clda parameter double; Cldr parameter double; Cm0 parameter double; Cma parameter double; Cmq parameter double; Cmadot parameter double; Cmu parameter double; Cmde parameter double; Cnb parameter double; Cnp parameter double; Cnr parameter double; Cnda parameter double; Cndr parameter double; xT0 parameter double; xT1 parameter double; xT2 parameter double; Ptrim parameter double; Qtrim parameter double; Rtrim parameter double; Utrim parameter double; Athrottle parameter double; Bthrottle parameter double; Aelevator parameter double; Belevator parameter double; Aaileron parameter double; Baileron parameter double; Arudder parameter double; Brudder parameter double; ThrottleMax parameter double; ThrottleMin parameter double; ElevatorMax parameter double; ElevatorMin parameter double; AileronMax parameter double; AileronMin parameter double; RudderMax parameter double; RudderMin parameter double
function [F,...
          falpha_un_o]...
           =...
          Jacobian_F(u,...
                     x_est,...
                     alphadot_o,...
                     dt,...
                     rho,...
                     S,Cbar,b,weight,g,IxxB,IyyB,IzzB,IxzB,...
                     CD0,CDu,CDa,CDq,CDadot,CDde,...
                     CD0_bar,...
                     Cyb,Cyp,Cyr,Cyda,Cydr,...
                     CL0,CLa,CLq,CLadot,CLu,CLde,...
                     Clb,Clp,Clr,Clda,Cldr,...
                     Cm0,Cma,Cmq,Cmadot,Cmu,Cmde,...
                     Cnb,Cnp,Cnr,Cnda,Cndr,...
                     xT0,xT1,xT2,...
                     Ptrim,Qtrim,Rtrim,Utrim,...
                     Athrottle,Bthrottle,...
                     Aelevator,Belevator,...
                     Aaileron,Baileron,...
                     Arudder,Brudder,...
                     ThrottleMax,ThrottleMin,...
                     ElevatorMax,ElevatorMin,...
                     AileronMax,AileronMin,...
                     RudderMax,RudderMin)
          
%#codegen

delta=0.00001;
M=zeros(15,15);

THL_o=x_est(1);
EL_o=x_est(2);
AIL_o=x_est(3);
RDR_o=x_est(4);
VT_o=x_est(5);
alpha_o=x_est(6);
beta_o=x_est(7);
phi_o=x_est(8);
theta_o=x_est(9);
psi_o=x_est(10);
P_o=x_est(11);
Q_o=x_est(12);
R_o=x_est(13);
alphab_o=x_est(14);
betab_o=x_est(15);

THLcmd_o=u(1);
ELcmd_o=u(2);
AILcmd_o=u(3);
RDRcmd_o=u(4);
accelX_meas_o=u(5);
accelY_meas_o=u(6);
accelZ_meas_o=u(7);

%unperturbed
[fTHL_un_o,fEL_un_o,fAIL_un_o,fRDR_un_o,...
 fVT_un_o,falpha_un_o,fbeta_un_o,fphi_un_o,ftheta_un_o,fpsi_un_o,fP_un_o,fQ_un_o,fR_un_o,...
 ~,~,...
 ~,~,~...
 ]...
 =f_x_u_state_EKF_sailplane(...
                    alphadot_o,...
                    THL_o,EL_o,AIL_o,RDR_o,...
                    VT_o,alpha_o,beta_o,phi_o,theta_o,psi_o,P_o,Q_o,R_o,...
                    alphab_o,betab_o,...
                    THLcmd_o,ELcmd_o,AILcmd_o,RDRcmd_o,...
                    accelX_meas_o,accelY_meas_o,accelZ_meas_o,...
                    rho,...
                    S,Cbar,b,weight,g,IxxB,IyyB,IzzB,IxzB,...
                    CD0,CDu,CDa,CDq,CDadot,CDde,...
                    CD0_bar,...
                    Cyb,Cyp,Cyr,Cyda,Cydr,...
                    CL0,CLa,CLq,CLadot,CLu,CLde,...
                    Clb,Clp,Clr,Clda,Cldr,...
                    Cm0,Cma,Cmq,Cmadot,Cmu,Cmde,...
                    Cnb,Cnp,Cnr,Cnda,Cndr,...
                    xT0,xT1,xT2,...
                    Ptrim,Qtrim,Rtrim,Utrim,...
                    Athrottle,Bthrottle,...
                    Aelevator,Belevator,...
                    Aaileron,Baileron,...
                    Arudder,Brudder,...
                    ThrottleMax,ThrottleMin,...
                    ElevatorMax,ElevatorMin,...
                    AileronMax,AileronMin,...
                    RudderMax,RudderMin);

f_x_un=[fTHL_un_o;fEL_un_o;fAIL_un_o;fRDR_un_o;...
        fVT_un_o;falpha_un_o;fbeta_un_o;fphi_un_o;ftheta_un_o;fpsi_un_o;fP_un_o;fQ_un_o;fR_un_o];
 
%perturbed
for i=1:13
    [fTHL_per_o,fEL_per_o,fAIL_per_o,fRDR_per_o,...
     fVT_per_o,falpha_per_o,fbeta_per_o,fphi_per_o,ftheta_per_o,fpsi_per_o,fP_per_o,fQ_per_o,fR_per_o,...
     ~,~,...
     ~,~,~...
     ]...
     =f_x_u_state_EKF_sailplane(...
                    alphadot_o,...
                    THL_o+delta*(i==1),EL_o+delta*(i==2),AIL_o+delta*(i==3),RDR_o+delta*(i==4),...
                    VT_o+delta*(i==5),alpha_o+delta*(i==6),beta_o+delta*(i==7),...
                    phi_o+delta*(i==8),theta_o+delta*(i==9),psi_o+delta*(i==10),...
                    P_o+delta*(i==11),Q_o+delta*(i==12),R_o+delta*(i==13),...
                    alphab_o,betab_o,...
                    THLcmd_o,ELcmd_o,AILcmd_o,RDRcmd_o,...
                    accelX_meas_o,accelY_meas_o,accelZ_meas_o,...
                    rho,...
                    S,Cbar,b,weight,g,IxxB,IyyB,IzzB,IxzB,...
                    CD0,CDu,CDa,CDq,CDadot,CDde,...
                    CD0_bar,...
                    Cyb,Cyp,Cyr,Cyda,Cydr,...
                    CL0,CLa,CLq,CLadot,CLu,CLde,...
                    Clb,Clp,Clr,Clda,Cldr,...
                    Cm0,Cma,Cmq,Cmadot,Cmu,Cmde,...
                    Cnb,Cnp,Cnr,Cnda,Cndr,...
                    xT0,xT1,xT2,...
                    Ptrim,Qtrim,Rtrim,Utrim,...
                    Athrottle,Bthrottle,...
                    Aelevator,Belevator,...
                    Aaileron,Baileron,...
                    Arudder,Brudder,...
                    ThrottleMax,ThrottleMin,...
                    ElevatorMax,ElevatorMin,...
                    AileronMax,AileronMin,...
                    RudderMax,RudderMin);

          f_x_per=[fTHL_per_o;fEL_per_o;fAIL_per_o;fRDR_per_o;...
                   fVT_per_o;falpha_per_o;fbeta_per_o;fphi_per_o;ftheta_per_o;fpsi_per_o;fP_per_o;fQ_per_o;fR_per_o];
               
          M(1:13,i)=(f_x_per-f_x_un)/delta;
end;
      
%F=expm(dt*M);            
F=eye(15)+(dt*M)+1/2*(dt*M)^2+1/6*(dt*M)^3+1/24*(dt*M)^4; %approximate exponential

== matlab function State Observer/EKF/K[k] (states)/K_[k]/Transpose ==
  data: u input double; HT_k output double
function HT_k = fcn(u)
%#codegen

HT_k = u';

== matlab function State Observer/EKF/K[k] (states)/Transpose ==
  data: u input double; FT_k_1 output double
function FT_k_1 = fcn(u)
%#codegen

FT_k_1=u';

== matlab function State Observer/EKF/K[k] (states)/Jacobian H ==
  data: unused input double; H output double; x_est input double; HN0noaa parameter double; HE0noaa parameter double; HD0noaa parameter double
function H...
          =...
          Jacobian_H(~,...
                     x_est,...
                     HN0noaa,HE0noaa,HD0noaa)          
%#codegen

delta=0.00001;
H=zeros(9,15);

THL_o=x_est(1);
EL_o=x_est(2);
AIL_o=x_est(3);
RDR_o=x_est(4);
VT_o=x_est(5);
alpha_o=x_est(6);
beta_o=x_est(7);
phi_o=x_est(8);
theta_o=x_est(9);
psi_o=x_est(10);
P_o=x_est(11);
Q_o=x_est(12);
R_o=x_est(13);
alphab_o=x_est(14);
betab_o=x_est(15);

%unperturbed
[hVT_un_o,halpha_un_o,hbeta_un_o,hP_un_o,hQ_un_o,hR_un_o,...
 hHxbody_un_o,hHybody_un_o,hHzbody_un_o...
 ]...
 =h_x_u_state_EKF_sailplane(...
                            THL_o,EL_o,AIL_o,RDR_o,...
                            VT_o,alpha_o,beta_o,phi_o,theta_o,psi_o,P_o,Q_o,R_o,...
                            alphab_o,betab_o,...
                            HN0noaa,HE0noaa,HD0noaa);

h_x_un=[hVT_un_o,halpha_un_o,hbeta_un_o,hP_un_o,hQ_un_o,hR_un_o,...
        hHxbody_un_o,hHybody_un_o,hHzbody_un_o];
 
%perturbed
for i=1:15
    [hVT_per_o,halpha_per_o,hbeta_per_o,hP_per_o,hQ_per_o,hR_per_o,...
     hHxbody_per_o,hHybody_per_o,hHzbody_per_o...
     ]...
     =h_x_u_state_EKF_sailplane(...
                    THL_o+delta*(i==1),EL_o+delta*(i==2),AIL_o+delta*(i==3),RDR_o+delta*(i==4),...
                    VT_o+delta*(i==5),alpha_o+delta*(i==6),beta_o+delta*(i==7),...
                    phi_o+delta*(i==8),theta_o+delta*(i==9),psi_o+delta*(i==10),...
                    P_o+delta*(i==11),Q_o+delta*(i==12),R_o+delta*(i==13),...
                    alphab_o+delta*(i==14),betab_o+delta*(i==15),...
                    HN0noaa,HE0noaa,HD0noaa);
          h_x_per=[hVT_per_o,halpha_per_o,hbeta_per_o,hP_per_o,hQ_per_o,hR_per_o,...
                   hHxbody_per_o,hHybody_per_o,hHzbody_per_o];
               
          H(1:9,i)=(h_x_per-h_x_un)/delta;
end;
